simulink model "rtwdemo_secondOrderSystem"  (R2022a)
settings: Solver=FixedStepAuto  StartTime=0.0  StopTime=1  FixedStep=0.001  RelTol=1e-3  EnableMultiTasking=on
settings Model: PacingRate=0.010000  Creator=The MathWorks, Inc.  LastModifiedBy=DNE
settings SolverCC: AlgebraicLoopSolver=TrustRegion
settings DataIOCC: SaveFormat=StructureWithTime  SaveState=on  InspectSignalLogs=on  ReturnWorkspaceOutputs=off
settings OptimizationCC: OptimizeBlockIOStorage=off  BufferReuse=off  GlobalBufferReuse=off  ExpressionFolding=off  ExpressionDepthLimit=2147483647  LocalBlockOutputs=off  InitFltsAndDblsToZero=on  LifeSpan=inf  OptimizeDataStoreBuffers=off  BusAssignmentInplaceUpdate=off
settings DebuggingCC: SaveWithParameterizedLinksMsg=none  CheckExecutionContextPreStartOutputMsg=on  SignalResolutionControl=TryResolveAllWithWarning  MultiTaskDSMMsg=warning  MultiTaskCondExecSysMsg=none  UnconnectedInputMsg=warning  UnconnectedOutputMsg=warning  UnconnectedLineMsg=warning  AllowSymbolicDim=off  StateNameClashWarn=warning  SFUnexpectedBacktrackingDiag=warning  SFNoUnconditionalDefaultTransitionDiag=warning  SFExecutionAtInitializationDiag=none  SFMachineParentedDataDiag=warning  ArithmeticOperatorsInVariantConditions=warning
settings ModelReferenceCC: PropagateSignalLabelsOutOfModel=off
settings SFSimCC: SimUseLocalCustomCode=off
settings RTWCC: Description=Generic Real-Time Target  GenerateReport=on  RTWVerbose=off  RTWUseLocalCustomCode=off  BuildConfiguration=Debug  LaunchReport=on  DLArmComputeVersion=19.05
settings CodeAppCC: ForceParamTrailComments=on  MATLABSourceComments=on  EnableCustomComments=on
settings GRTTargetCC: TargetLangStandard=C89/C90 (ANSI)  UtilityFuncGeneration=Shared location  CombineSignalStateStructs=on  MatFileLogging=off  SupportVariableSizeSignals=on  ExtMode=on  ExtModeStaticAlloc=on  ExtModeTransport=2  ExtModeMexFile=ext_xcp  ExtModeIntrfLevel=Level2 - Open  MultiInstanceErrorCode=Warning
settings ConfigComp: CovMetricSettings=dw  CovSaveCumulativeToWorkspaceVar=on  CovSaveSingleToWorkspaceVar=on  CovExternalEMLEnable=off

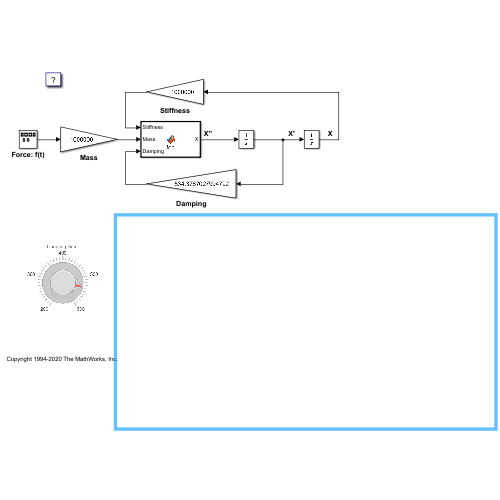
[thumbnail: Simulink's stored preview of the top-level diagram]
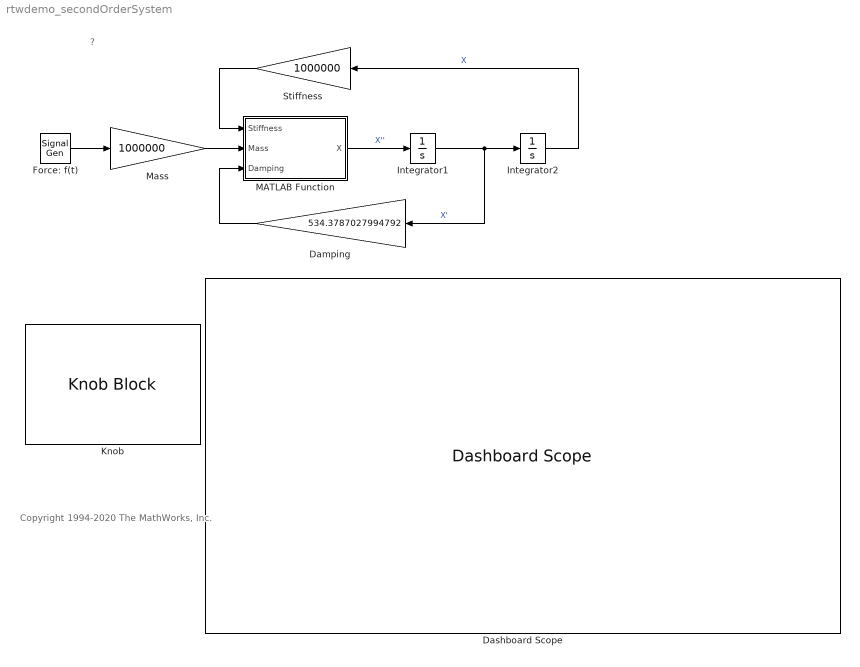
== system rtwdemo_secondOrderSystem ==
  note: Copyright 1994-2020 The MathWorks, Inc.
  note: ?
  Damping : Gain  Gain=534.3787027994792  SaturateOnIntegerOverflow=on  OutDataTypeStr=Inherit: Same as input  ParamDataTypeStr=Inherit: Same as input
  Dashboard Scope : DashboardScope  TimeSpan=0.20000000000000001  Ymin=-10  Ymax=10
  Force: f(t) : SignalGenerator  WaveForm=square  Amplitude=4  Frequency=20
  Integrator1 : Integrator
  Integrator2 : Integrator
  Knob : KnobBlock  ScaleMin=200  ScaleMax=600  TickInterval=100
  MATLAB Function : MATLAB Function  TreatAsAtomicUnit=on
  Mass : Gain  Gain=1000000  SaturateOnIntegerOverflow=on  OutDataTypeStr=Inherit: Same as input  ParamDataTypeStr=Inherit: Same as input
  Stiffness : Gain  Gain=1000000  SaturateOnIntegerOverflow=on  OutDataTypeStr=Inherit: Same as input  ParamDataTypeStr=Inherit: Same as input
  wires:
  Integrator1/1 -> Integrator2/1, Damping/1  "X'"
  Integrator2/1 -> Stiffness/1  "X"
  Damping/1 -> MATLAB Function/3(Damping)
  MATLAB Function/1(X) -> Integrator1/1  "X''"
  Force: f(t)/1 -> Mass/1
  Stiffness/1 -> MATLAB Function/1(Stiffness)
  Mass/1 -> MATLAB Function/2(Mass)

== matlab function rtwdemo_secondOrderSystem/MATLAB Function ==
  data: Stiffness input; X output; Mass input; Damping input
function X = fcn(Stiffness,Mass,Damping)

X = (-Stiffness+Mass-Damping);
